simulink model "BatteryTesting100"  (R2022a)
settings: Solver=ode23tb  StartTime=0.0  StopTime=inf  RelTol=1e-3  EnableMultiTasking=on
undefined symbols (not defined in the file or in its folder): Batt, Battery, BatteryCback, BatteryLoadFcn, DC, DOD, gcbh, Q, sps_rtmsupport, spsBatteryLib, Temp
libraries: simulink x7, spsControlledVoltageSourceLib x1, spsCurrentMeasurementLib x1, spsBatteryModel x1, simulink_extras x1, spsSeriesRLCBranchLib x1, spsControlledCurrentSourceLib x1, spspowerguiLib x1
settings Model: Creator=MathWorks  LastModifiedBy=awesomezhao
settings SolverCC: AlgebraicLoopSolver=TrustRegion
settings DataIOCC: LimitDataPoints=on  ReturnWorkspaceOutputs=off
settings OptimizationCC: LifeSpan=inf
settings DebuggingCC: UnconnectedInputMsg=warning  UnconnectedOutputMsg=warning  UnconnectedLineMsg=warning  AllowSymbolicDim=off  SFUnexpectedBacktrackingDiag=warning  SFNoUnconditionalDefaultTransitionDiag=warning  SFExecutionAtInitializationDiag=none  SFMachineParentedDataDiag=warning  ArithmeticOperatorsInVariantConditions=warning
settings HardwareCC: ProdBitPerPointer=32  ProdBitPerSizeT=32  ProdBitPerPtrDiffT=32  ProdLargestAtomicFloat=None  ProdIntDivRoundTo=Undefined  ProdEndianess=Unspecified  ProdWordSize=32  ProdHWDeviceType=32-bit Generic
settings ModelReferenceCC: PropagateSignalLabelsOutOfModel=off
settings SFSimCC: SimUseLocalCustomCode=off  CustomCodeUndefinedFunction=UseInterfaceOnly
settings RTWCC: RTWUseLocalCustomCode=off  DLArmComputeVersion=19.05
settings CodeAppCC: StateflowObjectComments=on
settings GRTTargetCC: TargetLangStandard=C89/C90 (ANSI)
settings ConfigComp: CovMetricSettings=dw  CovSaveCumulativeToWorkspaceVar=on  CovSaveSingleToWorkspaceVar=on  CovExternalEMLEnable=off
settings SimscapeCC: SimscapeNormalizeSystem=off

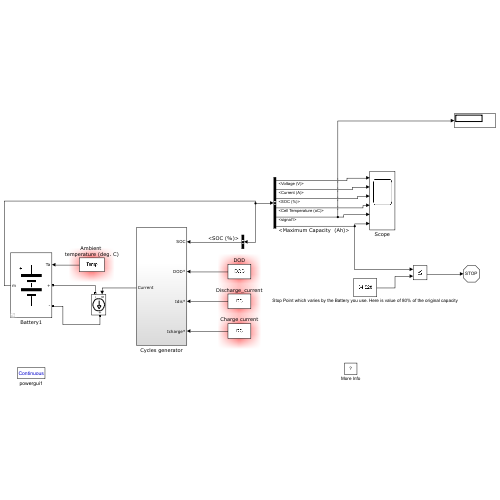
[thumbnail: Simulink's stored preview of the top-level diagram]
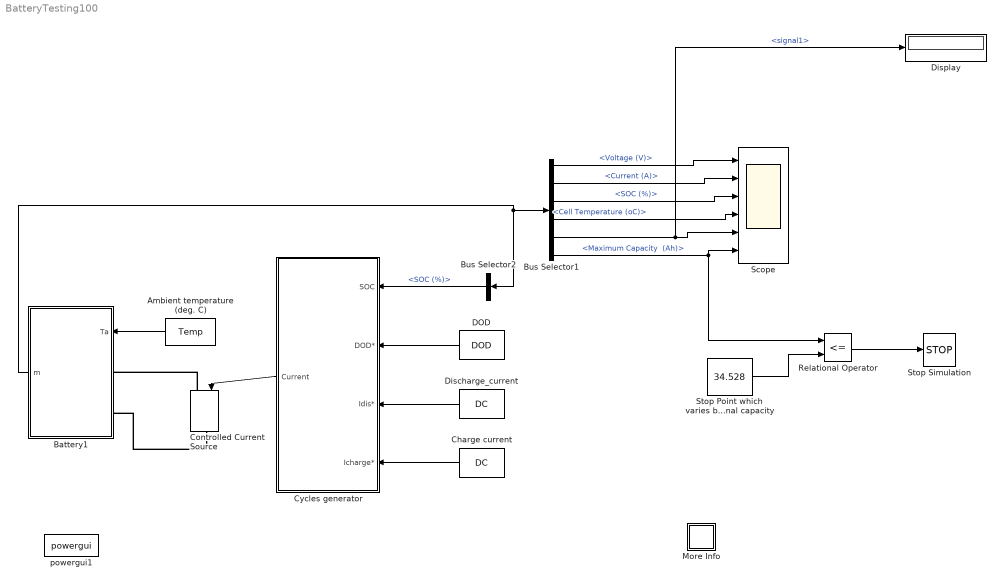
== system BatteryTesting100 ==
  Ambient temperature (deg. C) : Constant  Value=Temp
  Battery1 : Subsystem  AncestorBlock=spsBatteryLib/Battery  DialogController=POWERSYS.PowerSysDialog  LoadFcn=sps_rtmsupport('LoadFcn',gcbh); BatteryLoadFcn(gcb)  InitFcn=BatteryCback(gcb,1)  StartFcn=sps_rtmsupport('StartFcn',gcbh);  StopFcn=sps_rtmsupport('StopFcn',gcbh);  mask(Battery){BatType=Lithium-Ion, ShowTempParam=on, ThermalPreset=12.8V  40Ah  (LiFeMgPO4), ShowAgeParam=on, NomV=12.6, NomQ=40, SOC=100, Batt_Tr=90, PresetModel=off, MaxQ=40, MinV=10.5, FullV=13.8, Dis_rate=20, R=0.015, Normal_OP=30.14, expZone=[13.1          0.5], current=[0.15 1.3 3.25], Units=Ampere-hour, Tci=25, NomT=20, T2=0, MaxQ2=36, FullV2=13, Normal_OP2=11.7, expZone2=[12.67            4], Rca=0.6411, ti=4880, Dp=0, Neq0=0, Tsim=30, Ta1=23, Qeol=40*0.9, Reol=0.0126*1.2, Char_age=[20, 80], Dis_age=[20, 80], N1=1500, N2=10445, N3=1017, N4=1460, Ta2=45, N5=982}
      mask prompts: BatType "Type:"; ShowTempParam "Simulate temperature effects"; ThermalPreset "Use a preset battery:"; ShowAgeParam "Simulate aging effects"; NomV "Nominal voltage (V)"; NomQ "Rated capacity (Ah)"; SOC "Initial state-of-charge (%)"; Batt_Tr "Battery response time (s)"; PresetModel "Determined from the nominal parameters of the battery"; MaxQ "Maximum capacity (Ah)"; MinV "Cut-off Voltage (V)"; FullV "Fully charged voltage (V)"; Dis_rate "Nominal discharge current (A)"; R "Internal resistance (Ohms)"; Normal_OP "Capacity (Ah) at nominal voltage"; expZone "Exponential zone [Voltage (V), Capacity (Ah)]"; current "Discharge current [i1, i2, i3,...] (A)"; Tci "Initial cell temperature (deg. C)"; NomT "Nominal ambient temperature T1 (deg. C)"; T2 "Second ambient temperature T2 (deg. C)"; MaxQ2 "Maximum capacity (Ah)"; FullV2 "Initial discharge voltage (V)"; Normal_OP2 "Voltage at 90% maximum capacity (V)"; expZone2 "Exponential zone [Voltage (V), Capacity (Ah)]"; Rca "Thermal resistance, cell-to-ambient (deg. C/W)"; ti "Thermal time constant, cell-to-ambient (s)"; Dp "Heat loss difference [charge vs. discharge] (W)"; Neq0 "Initial battery age (Equivalent full cycles)"; Tsim "Aging model sampling time (s)"; Ta1 "Ambient temperature Ta1 (deg. C)"; Qeol "Capacity at EOL (End Of Life) (Ah)"; Reol "Internal resistance at EOL (Ohms)"; Char_age "Charge current (nominal, maximum) [Ic (A), Icmax (A)]"; Dis_age "Discharge current (nominal, maximum) [Id (A), Idmax (A)]"; N1 "Cycle life at 100 % DOD, Ic and Id (Cycles)"; N2 "Cycle life at 25 % DOD, Ic and Id (Cycles)"; N3 "Cycle life at 100 % DOD, Ic and Idmax (Cycles)"; N4 "Cycle life at 100 % DOD, Icmax and Id (Cycles)"; Ta2 "Ambient temperature Ta2 (deg. C)"; N5 "Cycle life at 100 % DOD, Ic and Id (Cycles)"
      mask help: Implements a generic battery model for most popular battery types. Temperature and aging (due to cycling) effects can be specified for Lithium-Ion battery type.
      mask init:
      | block = gcb;
      | BatteryCback(block,3)
      | [Batt BT, WantBlockChoice, Ts] = BatteryParam(NomV,NomQ,MaxQ,MinV,FullV,Dis_rate,R,Normal_OP,expZone,block,0);
      | powericon('SetInternalModels','set',block,WantBlockChoice);
      | BatteryCback(block,1);
      settings: CopyFcn=sps_rtmsupport('CopyFcn',gcbh);  DeleteFcn=sps_rtmsupport('DeleteFcn',gcbh);  UndoDeleteFcn=sps_rtmsupport('UndoDeleteFcn',gcbh);  ModelCloseFcn=sps_rtmsupport('ModelCloseFcn',gcbh);  PreSaveFcn=sps_rtmsupport('PreSaveFcn',gcbh);  PostSaveFcn=sps_rtmsupport('PostSaveFcn',gcbh);  NameChangeFcn=sps_rtmsupport('NameChangeFcn',gcbh);  PreCopyFcn=sps_rtmsupport('PreCopyFcn',gcbh);  OpenFcn=sps_rtmsupport('OpenFcn',gcbh, [1,2,3,4,9,18]);  CloseFcn=sps_rtmsupport('CloseFcn',gcbh);  PreDeleteFcn=sps_rtmsupport('PreDeleteFcn',gcbh);
      mask Help: helpview(psbhelp)
      mask TypeOptions BatType: Lead-Acid | Lithium-Ion | Nickel-Cadmium | Nickel-Metal-Hydride
      mask Callback BatType: BatteryCback(gcb,1)
      mask Callback ShowTempParam: BatteryCback(gcb,1)
      mask TypeOptions ThermalPreset: no | 3.3V  2.3Ah  (LiFePO4) | 3.6V  2050mAh   (LiCoO2) | 3.6V  2.0Ah | 3.6V  3.6Ah  (LiNiO2) | 3.6V  4.5Ah | 3.6V  48Ah  (LiNiO2) | 3.7V  4.4Ah | 7.4V  5.4Ah  (LiCoO2) | 11.1V  6600mAh  (LiCoO2) | 12.8V  40Ah  (LiFeMgPO4)
      mask Callback ThermalPreset: BatteryCback(gcb,4)
      mask Callback ShowAgeParam: BatteryCback(gcb,1)
      mask Callback PresetModel: BatteryCback(gcb,1)
      mask TypeOptions Units: Ampere-hour | Time
      mask Callback ti: sps_rtmsupport('parametereditingmodes',gcbh, [1,2,3,4,9,18]);
      mask DialogControl ParameterTabVar0 Prompt: Parameters
      mask DialogControl Tempcontainer Prompt: Temperature
      mask DialogControl Agecontainer Prompt: Aging
      mask DialogControl ParameterTabVar01 Prompt: Discharge
      mask DialogControl Container9 Prompt: Display characteristics
      mask DialogControl PlotButton Prompt: Plot
      mask DialogControl PlotButton Callback: BatteryCback(gcb,0)
      mask DialogControl Temperature Prompt: Temperature
      mask DialogControl Container7 Prompt: Discharge parameters at T2
      mask DialogControl Container8 Prompt: Thermal response and Heat loss
      mask DialogControl Aging Prompt: Aging
      mask DialogControl Container16 Prompt: Aging characteristics at ambient temperature Ta1
      mask DialogControl Container13 Prompt: Aging characteristics at ambient temperature Ta2
  Bus Selector1 : BusSelector  OutputSignals="Voltage (V),Current (A),SOC (%),Cell Temperature (oC),signal1,Maximum Capacity  (Ah)"
  Bus Selector2 : BusSelector  OutputSignals=SOC (%)
  Charge current : Constant  Value=DC
  Controlled Current Source : spsControlledCurrentSourceLib/Controlled Current Source  Initialize=on  Source_Type=AC  Amplitude=0  Phase=0  Frequency=0  Measurements=None
  Cycles generator : Subsystem
  DOD : Constant  Value=DOD
  Discharge_current : Constant  Value=DC
  Display : Display
  More Info : Subsystem
      settings: OpenFcn=showdemo(bdroot(gcb))
      mask Display: disp('?')
  Relational Operator : RelationalOperator  Operator=<=  OutDataTypeStr=boolean  RndMeth=Simplest  InputSameDT=off
  Scope : Scope  NumInputPorts=6
  Stop Point which varies by the Battery you use. Here is value of 80% of the original capacity : Constant  Value=34.528
  Stop Simulation : Stop
  powergui1 : spspowerguiLib/powergui  SimulationMode=Continuous  SampleTime=36  frequency=60  Iterations=50  frequencyindice=0  Pbase=100e6  ErrMax=1e-4  UnitsV=kV  UnitsW=MW  buscounter=0  FunctionMessages=off  echomessages=off  EnableUseOfTLC=off  CurrentSourceSwitches=on  DisableSnubberDevices=off  DisableRonSwitches=off  DisableVfSwitches=off  DisplayEquations=off  AutomaticDiscreteSolvers=off  SolverType=Tustin  Interpol=off  ExternalGateDelay=off  methode=off  Ts=0  x0status=blocks  SPID=off  SwTol=0  HookPort=off  NonlinearTolerance=1e-4  nMaxIteration=100  ContinueOnMaxIteration=off  RestoreLinks=warning  ResistiveCurrentMeasurement=off  Frange=[0:2:500]  Ylog=off  Xlog=on  ShowGrid=off  save=off  variable=ZData  structure=0  ZoomFFT=on  StartTime=0.0  cycles=1  DisplayStyle=1  fundamental=60  FreqAxis=off  MaxFrequency=1000  frequencyindicesteady=1  RmsSteady=1  display=off
  wires:
  Ambient temperature (deg. C)/1 -> Battery1/1(Ta)
  Battery1/1(m) -> Bus Selector2/1, Bus Selector1/1
  Bus Selector1/6 -> Scope/6, Relational Operator/1  "<Maximum Capacity  (Ah)>"
  Cycles generator/1(Current) -> Controlled Current Source/1
  Bus Selector2/1 -> Cycles generator/1(SOC)  "<SOC (%)>"
  Charge current/1 -> Cycles generator/4(Icharge*)
  DOD/1 -> Cycles generator/2(DOD*)
  Discharge_current/1 -> Cycles generator/3(Idis*)
  Stop Point which varies by the Battery you use. Here is value of 80% of the original capacity/1 -> Relational Operator/2
  Relational Operator/1 -> Stop Simulation/1
  Bus Selector1/1 -> Scope/1  "<Voltage (V)>"
  Bus Selector1/2 -> Scope/2  "<Current (A)>"
  Bus Selector1/3 -> Scope/3  "<SOC (%)>"
  Bus Selector1/4 -> Scope/4  "<Cell Temperature (oC)>"
  Bus Selector1/5 -> Display/1, Scope/5  "<signal1>"
  connections:
  Controlled Current Source/LConn1 -- Battery1/LConn1
  Controlled Current Source/RConn1 -- Battery1/LConn2

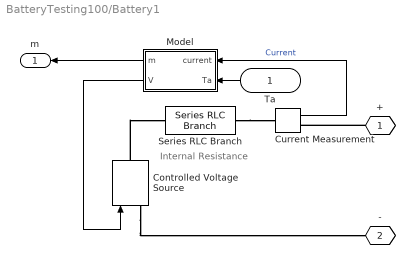
== system BatteryTesting100/Battery1 ==
  note: Internal Resistance
  Ta : Inport
  Controlled Voltage Source : spsControlledVoltageSourceLib/Controlled Voltage Source  Initialize=on  Source_Type=AC  Amplitude=0  Phase=0  Frequency=0  Measurements=None
  Current Measurement : spsCurrentMeasurementLib/Current Measurement  PhasorSimulation=off  OutputType=Complex  PSBequivalent=0
  Model : Subsystem  AncestorBlock=spsBatteryModel/Continuous thermal aging
  Series RLC Branch : spsSeriesRLCBranchLib/Series RLC Branch  LConnTagsString=__new0  RConnTagsString=__new0  BranchType=R  Resistance=Batt.R  Inductance=1e-3  SetiL0=off  InitialCurrent=0  Capacitance=1e-6  Setx0=off  InitialVoltage=0  Measurements=None
  + : PMIOPort  Tag=PMCPort  Side=Left
  - : PMIOPort  Tag=PMCPort  Port=2  Side=Left
  m : Outport  VectorParamsAs1DForOutWhenUnconnected=off
  wires:
  Model/2(V) -> Controlled Voltage Source/1
  Model/1(m) -> m/1
  Current Measurement/1 -> Model/1(current)  "Current"
  Ta/1 -> Model/2(Ta)
  connections:
  +/RConn1 -- Current Measurement/RConn1
  Controlled Voltage Source/LConn1 -- -/RConn1
  Controlled Voltage Source/RConn1 -- Series RLC Branch/LConn1
  Series RLC Branch/RConn1 -- Current Measurement/LConn1

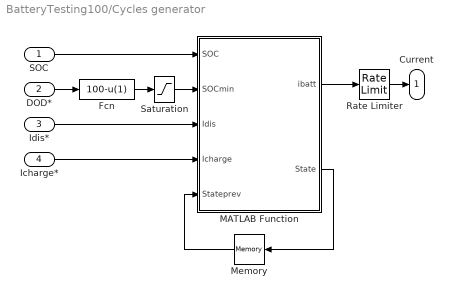
== system BatteryTesting100/Cycles generator ==
  SOC : Inport
  DOD* : Inport  Port=2
  Idis* : Inport  Port=3
  Icharge* : Inport  Port=4
  Fcn : Fcn  Expr=100-u(1)
  MATLAB Function : MATLAB Function  TreatAsAtomicUnit=on
  Memory : Memory  InitialCondition=1
  Rate Limiter : RateLimiter  RisingSlewLimit=1000  FallingSlewLimit=-1000  SampleTimeMode=inherited
  Saturation : Saturate  UpperLimit=98  LowerLimit=1
  Current : Outport  VectorParamsAs1DForOutWhenUnconnected=off
  wires:
  MATLAB Function/1(ibatt) -> Rate Limiter/1
  SOC/1 -> MATLAB Function/1(SOC)
  Memory/1 -> MATLAB Function/5(Stateprev)
  MATLAB Function/2(State) -> Memory/1
  DOD*/1 -> Fcn/1
  Fcn/1 -> Saturation/1
  Saturation/1 -> MATLAB Function/2(SOCmin)
  Idis*/1 -> MATLAB Function/3(Idis)
  Icharge*/1 -> MATLAB Function/4(Icharge)
  Rate Limiter/1 -> Current/1

== system BatteryTesting100/More Info ==

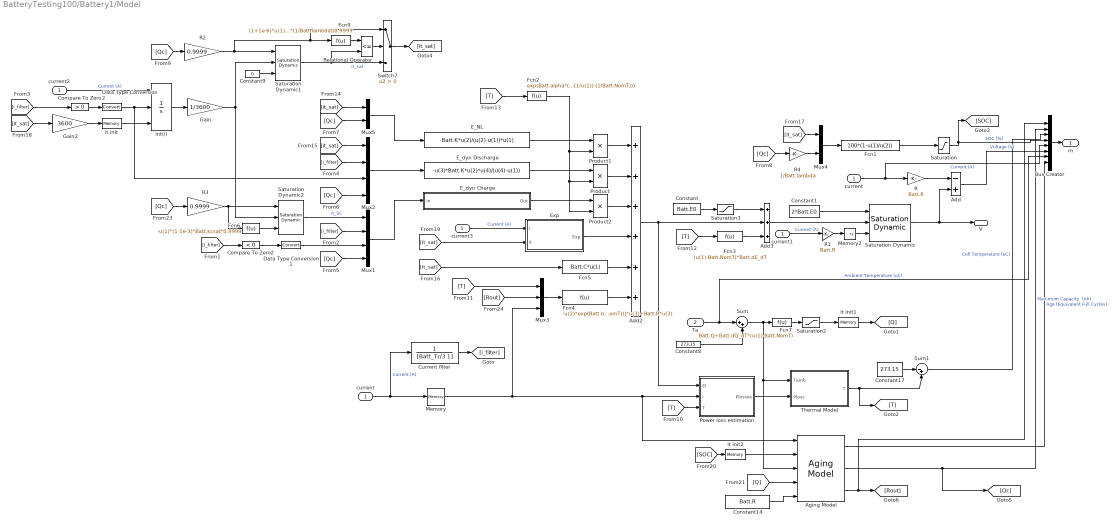
== system BatteryTesting100/Battery1/Model ==
  current : Inport
  Ta : Inport  Port=2
  Add : Sum  Inputs=-+
  Add2 : Sum  Inputs=++++++
  Add3 : Sum  Inputs=+++
  Aging Model : spsBatteryModel/Aging Model  SystemSampleTime=-1  VariantActivationTime=update diagram  Latency=0  AutoFrameSizeCalculation=off
      settings: SourceProductBaseCode=PS
  Bus Creator : BusCreator  Inputs=8
  Compare To Zero : simulink/Logic and Bit Operations/Compare To Zero  relop=>  OutDataTypeStr=uint8
  Compare To Zero2 : simulink/Logic and Bit Operations/Compare To Zero  relop=<  OutDataTypeStr=uint8
  Constant : Constant  Value=Batt.E0
  Constant1 : Constant  Value=2*Batt.E0
  Constant14 : Constant  Value=Batt.R
  Constant17 : Constant  Value=273.15
  Constant8 : Constant  Value=273.15
  Constant9 : Constant  Value=0
  Current filter : TransferFcn  Denominator=[Batt_Tr/3 1]
  Data Type Conversion1 : DataTypeConversion  SaturateOnIntegerOverflow=off  RndMeth=Floor
  Data Type Conversion2 : DataTypeConversion  SaturateOnIntegerOverflow=off  RndMeth=Floor
  E_NL : Fcn  Expr=-Batt.K*u(2)/(u(2)-u(1))*u(1)
  E_dyn Charge : Subsystem
  E_dyn Discharge : Fcn  Expr=-u(3)*Batt.K*u(2)*u(4)/(u(4)-u(1))
  Exp : Subsystem
  Fcn1 : Fcn  Expr=100*(1-u(1)/u(2))
  Fcn2 : Fcn  Expr=exp(Batt.alpha*((1/u(1))-(1/Batt.NomT)))
  Fcn3 : Fcn  Expr=(u(1)-Batt.NomT)*Batt.dE_dT
  Fcn4 : Fcn  Expr=-u(2)*exp(Batt.beta*((1/u(1))-(1/Batt.NomT)))*u(3)+Batt.R*u(3)
  Fcn5 : Fcn  Expr=-Batt.C*u(1)
  Fcn6 : Fcn  Expr=-u(1)*(1-1e-3)*Batt.kcsat*0.9999
  Fcn7 : Fcn  Expr=Batt.Q+Batt.dQ_dT*(u(1)-Batt.NomT)
  Fcn9 : Fcn  Expr=(1+1e-6)*u(1)*(1/Batt.lambda)/0.9999
  Gain : Gain  Gain=1/3600
  Gain2 : Gain  Gain=3600
  Memory : Memory
  Memory2 : Memory  InheritSampleTime=on
  Mux1 : Mux
  Mux2 : Mux
  Mux3 : Mux  Inputs=3
  Mux4 : Mux  Inputs=2
  Mux5 : Mux  Inputs=2
  Power loss estimation : Subsystem
  Product : Product
  Product1 : Product
  Product2 : Product
  R : Gain  Gain=Batt.R
  R1 : Gain  Gain=Batt.R
  R2 : Gain  Gain=0.9999
  R3 : Gain  Gain=0.9999
  R4 : Gain  Gain=1/Batt.lambda
  Relational Operator : RelationalOperator  Operator=<=  RndMeth=Simplest  InputSameDT=off
  Saturation : Saturate  UpperLimit=100  LowerLimit=0
  Saturation Dynamic : simulink/Discontinuities/Saturation Dynamic  OutMin=[]  OutMax=[]  OutDataTypeStr=Inherit: Same as second input  OutDataType=sfix(16)  OutScaling=2^-10  DoSatur=off
  Saturation Dynamic1 : simulink/Discontinuities/Saturation Dynamic  OutMin=[]  OutMax=[]  OutDataTypeStr=Inherit: Same as second input  OutDataType=sfix(16)  OutScaling=2^-10  DoSatur=off
  Saturation Dynamic2 : simulink/Discontinuities/Saturation Dynamic  OutMin=[]  OutMax=[]  OutDataTypeStr=Inherit: Same as second input  OutDataType=sfix(16)  OutScaling=2^-10  DoSatur=off
  Saturation2 : Saturate  UpperLimit=max(NomQ,Batt.Q)  LowerLimit=0
  Saturation3 : Saturate  UpperLimit=Batt.Va-Batt.dE_dT*(Batt.Tci-Batt.NomT)-Batt.A  LowerLimit=-inf
  Sum : Sum  Inputs=|++
  Sum1 : Sum  Inputs=|-+
  Switch7 : Switch  Criteria=u2 > Threshold  SaturateOnIntegerOverflow=off  InputSameDT=off
  Thermal Model : Subsystem  VariantControl=Continuous
  "current " : InportShadow
  current1 : InportShadow
  current2 : InportShadow
  current3 : InportShadow
  int(i) : Integrator  ExternalReset=rising  InitialConditionSource=external  InitialCondition=(1-SOC/100)*Q*3600  LimitOutput=on  UpperSaturationLimit=Batt.Qmax*3600
  it init : Memory  InitialCondition=(1-SOC/100)*Batt.Q*(1/Batt.lambda)*3600
  it init1 : Memory  InitialCondition=Batt.Q
  it init2 : Memory  InitialCondition=SOC
  m : Outport  VectorParamsAs1DForOutWhenUnconnected=off
  V : Outport  Port=2  VectorParamsAs1DForOutWhenUnconnected=off
  wires:
  Sum1/1 -> Bus Creator/3  "Cell Temperature (oC)"
  Thermal Model/1(T) -> [T], Sum1/2
  Constant17/1 -> Sum1/1
  Relational Operator/1 -> Switch7/2
  Fcn9/1 -> Relational Operator/1
  Switch7/1 -> [it_sat]
  R2/1 -> Saturation Dynamic1/1, Fcn9/1, Switch7/1
  Saturation Dynamic1/1 -> Switch7/3, Relational Operator/2  "it_sat"
  R1/1 -> Memory2/1
  Memory2/1 -> Saturation Dynamic/3
  current1/1 -> R1/1  "Current (A)"
  Constant9/1 -> Saturation Dynamic1/3
  Gain/1 -> Saturation Dynamic2/2, Saturation Dynamic1/2
  it init2/1 -> Aging Model/2
  [Rout] -> Mux3/2
  Aging Model/3 -> Bus Creator/1, [Rout]
  Constant14/1 -> Aging Model/5
  Aging Model/2 -> [Qc], Bus Creator/2  "Maximum Capacity  (Ah)"
  [Q] -> Aging Model/4
  [SOC] -> it init2/1
  [Qc] -> Mux5/2
  Saturation Dynamic/1 -> Add/2, V/1
  Saturation/1 -> [SOC], Bus Creator/4  "SOC (%)"
  R4/1 -> Mux4/2
  [T] -> Power loss estimation/3(T)
  Add2/1 -> Add3/2, Power loss estimation/1(El)
  R3/1 -> Saturation Dynamic2/1, Fcn6/1
  [Qc] -> R3/1
  [it_sat] -> Exp/2(it)
  [it_sat] -> Gain2/1
  [it_sat] -> Mux4/1
  [it_sat] -> Fcn5/1
  [it_sat] -> Mux2/1
  [it_sat] -> Mux5/1
  [T] -> Fcn2/1
  [T] -> Fcn3/1
  [T] -> Mux3/1
  [Qc] -> R2/1
  [Qc] -> R4/1
  [Qc] -> Mux2/4
  [Qc] -> Mux1/4
  it init1/1 -> [Q]
  [i_filter] -> Mux2/2
  [i_filter] -> Compare To Zero/1
  [i_filter] -> Mux1/2
  [i_filter] -> Compare To Zero2/1
  Current filter/1 -> [i_filter]
  "current "/1 -> Current filter/1, Memory/1  "Current (A)"
  current3/1 -> Exp/1(i)  "Current (A)"
  current2/1 -> int(i)/1  "Current (A)"
  Saturation2/1 -> it init1/1
  Saturation3/1 -> Add3/1
  Fcn7/1 -> Saturation2/1
  Sum/1 -> Fcn7/1, Thermal Model/1(Tamb), Aging Model/3
  Fcn6/1 -> Saturation Dynamic2/3
  Fcn3/1 -> Add3/3
  Mux5/1 -> E_NL/1
  Mux4/1 -> Fcn1/1
  Constant8/1 -> Sum/2
  Ta/1 -> Bus Creator/7, Sum/1  "Ambient Temperature (oC)"
  Fcn5/1 -> Add2/5
  Product2/1 -> Add2/3
  E_dyn Charge/1(Out) -> Product2/1
  Mux3/1 -> Fcn4/1
  Fcn4/1 -> Add2/6
  Fcn2/1 -> Product1/2, Product/2, Product2/2
  Power loss estimation/1(Plosses) -> Thermal Model/2(Ploss)
  Memory/1 -> Power loss estimation/2(i), Aging Model/1, Mux3/3
  Product1/1 -> Add2/1
  E_NL/1 -> Product1/1
  Product/1 -> Add2/2
  E_dyn Discharge/1 -> Product/1
  Add3/1 -> Saturation Dynamic/2
  Constant1/1 -> Saturation Dynamic/1
  Saturation Dynamic2/1 -> Mux1/1  "it_SC"
  Data Type Conversion1/1 -> Mux1/3
  Exp/1(Exp) -> Add2/4
  Gain2/1 -> it init/1
  Data Type Conversion2/1 -> int(i)/2, Mux2/3
  Compare To Zero2/1 -> Data Type Conversion1/1
  Compare To Zero/1 -> Data Type Conversion2/1
  it init/1 -> int(i)/3
  Mux1/1 -> E_dyn Charge/1(In)
  Constant/1 -> Saturation3/1
  Mux2/1 -> E_dyn Discharge/1
  Bus Creator/1 -> m/1
  R/1 -> Add/1
  Add/1 -> Bus Creator/6  "Voltage (V)"
  Fcn1/1 -> Saturation/1
  int(i)/1 -> Gain/1
  current/1 -> R/1, Bus Creator/5  "Current (A)"
  Aging Model/1 -> Bus Creator/8  "Age (Equivalent Full Cycles)"

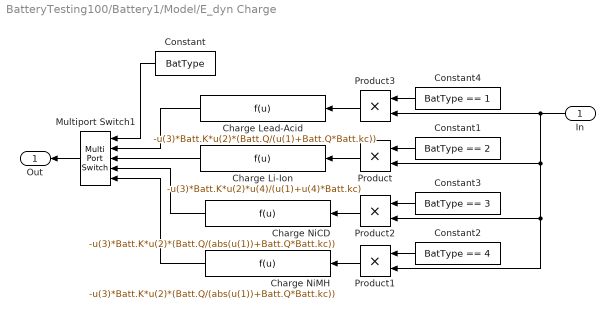
== system BatteryTesting100/Battery1/Model/E_dyn Charge ==
  In : Inport
  Charge Lead-Acid : Fcn  Expr=-u(3)*Batt.K*u(2)*(Batt.Q/(u(1)+Batt.Q*Batt.kc))
  Charge Li-Ion : Fcn  Expr=-u(3)*Batt.K*u(2)*u(4)/(u(1)+u(4)*Batt.kc)
  Charge NiCD : Fcn  Expr=-u(3)*Batt.K*u(2)*(Batt.Q/(abs(u(1))+Batt.Q*Batt.kc))
  Charge NiMH : Fcn  Expr=-u(3)*Batt.K*u(2)*(Batt.Q/(abs(u(1))+Batt.Q*Batt.kc))
  Constant : Constant  Value=BatType
  Constant1 : Constant  Value=BatType == 2  OutDataTypeStr=double
  Constant2 : Constant  Value=BatType == 4  OutDataTypeStr=double
  Constant3 : Constant  Value=BatType == 3  OutDataTypeStr=double
  Constant4 : Constant  Value=BatType == 1  OutDataTypeStr=double
  Multiport Switch1 : MultiPortSwitch  Inputs=4  SaturateOnIntegerOverflow=off  InputSameDT=off
  Product{,1..3} (4 alike) : Product  RndMeth=Zero
  Out : Outport  VectorParamsAs1DForOutWhenUnconnected=off
  wires:
  Constant4/1 -> Product3/1
  Product3/1 -> Charge Lead-Acid/1
  Constant3/1 -> Product2/1
  Product2/1 -> Charge NiCD/1
  Constant2/1 -> Product1/1
  Product1/1 -> Charge NiMH/1
  Constant1/1 -> Product/1
  Product/1 -> Charge Li-Ion/1
  In/1 -> Product2/2, Product1/2, Product/2, Product3/2
  Constant/1 -> Multiport Switch1/1
  Charge Lead-Acid/1 -> Multiport Switch1/2
  Charge NiCD/1 -> Multiport Switch1/4
  Charge NiMH/1 -> Multiport Switch1/5
  Charge Li-Ion/1 -> Multiport Switch1/3
  Multiport Switch1/1 -> Out/1

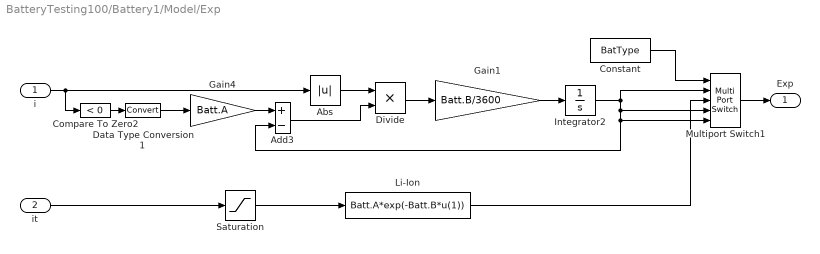
== system BatteryTesting100/Battery1/Model/Exp ==
  i : Inport
  it : Inport  Port=2
  Abs : Abs  SaturateOnIntegerOverflow=off
  Add3 : Sum  Inputs=+-
  Compare To Zero2 : simulink/Logic and Bit Operations/Compare To Zero  relop=<  OutDataTypeStr=uint8
  Constant : Constant  Value=BatType
  Data Type Conversion1 : DataTypeConversion  SaturateOnIntegerOverflow=off  RndMeth=Floor
  Divide : Product  Inputs=**
  Gain1 : Gain  Gain=Batt.B/3600
  Gain4 : Gain  Gain=Batt.A
  Integrator2 : Integrator  InitialCondition=Batt.A*exp(-Batt.B*(1-SOC/100)*Batt.Q)
  Li-Ion : Fcn  Expr=Batt.A*exp(-Batt.B*u(1))
  Multiport Switch1 : MultiPortSwitch  Inputs=4  SaturateOnIntegerOverflow=off  InputSameDT=off
  Saturation : Saturate  UpperLimit=Batt.Qmax*(1/Batt.lambda)  LowerLimit=-inf
  Exp : Outport  VectorParamsAs1DForOutWhenUnconnected=off
  wires:
  Saturation/1 -> Li-Ion/1
  Data Type Conversion1/1 -> Gain4/1
  Compare To Zero2/1 -> Data Type Conversion1/1
  Multiport Switch1/1 -> Exp/1
  Li-Ion/1 -> Multiport Switch1/3
  it/1 -> Saturation/1
  Constant/1 -> Multiport Switch1/1
  i/1 -> Compare To Zero2/1, Abs/1
  Gain1/1 -> Integrator2/1
  Add3/1 -> Divide/2
  Abs/1 -> Divide/1
  Divide/1 -> Gain1/1
  Gain4/1 -> Add3/1
  Integrator2/1 -> Multiport Switch1/5, Add3/2, Multiport Switch1/4, Multiport Switch1/2

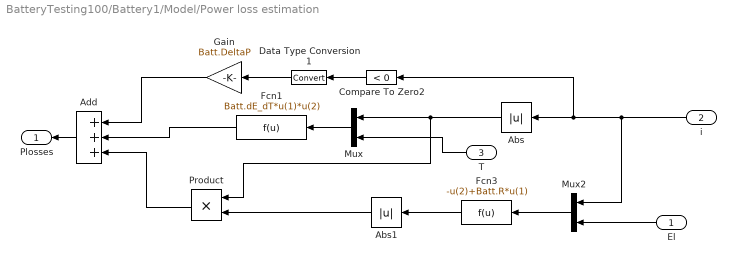
== system BatteryTesting100/Battery1/Model/Power loss estimation ==
  El : Inport
  i : Inport  Port=2
  T : Inport  Port=3
  Abs : Abs  SaturateOnIntegerOverflow=off
  Abs1 : Abs  SaturateOnIntegerOverflow=off
  Add : Sum  Inputs=+++
  Compare To Zero2 : simulink/Logic and Bit Operations/Compare To Zero  relop=<  OutDataTypeStr=uint8
  Data Type Conversion1 : DataTypeConversion  SaturateOnIntegerOverflow=off  RndMeth=Floor
  Fcn1 : Fcn  Expr=Batt.dE_dT*u(1)*u(2)
  Fcn3 : Fcn  Expr=-u(2)+Batt.R*u(1)
  Gain : Gain  Gain=Batt.DeltaP
  Mux : Mux  Inputs=2
  Mux2 : Mux  Inputs=2
  Product : Product
  Plosses : Outport  VectorParamsAs1DForOutWhenUnconnected=off
  wires:
  Gain/1 -> Add/1
  Data Type Conversion1/1 -> Gain/1
  Compare To Zero2/1 -> Data Type Conversion1/1
  Fcn1/1 -> Add/2
  Product/1 -> Add/3
  Mux2/1 -> Fcn3/1
  Fcn3/1 -> Abs1/1
  El/1 -> Mux2/2
  Abs1/1 -> Product/2
  Abs/1 -> Product/1, Mux/1
  Mux/1 -> Fcn1/1
  Add/1 -> Plosses/1
  T/1 -> Mux/2
  i/1 -> Mux2/1, Abs/1, Compare To Zero2/1

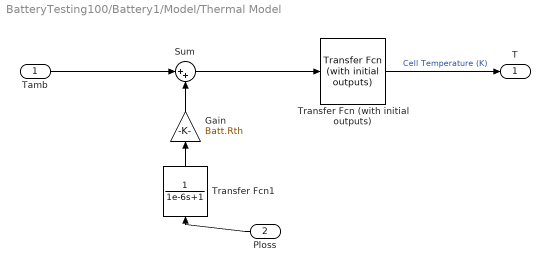
== system BatteryTesting100/Battery1/Model/Thermal Model ==
  Tamb : Inport
  Ploss : Inport  Port=2
  Gain : Gain  Gain=Batt.Rth
  Sum : Sum  Inputs=|++
  Transfer Fcn (with initial outputs) : simulink_extras/Additional Linear/Transfer Fcn (with initial outputs)  N=[1]  D="[Batt.tc  1]"  Y0=Batt.Tci  U0=0
  Transfer Fcn1 : TransferFcn  Denominator=[1e-6 1]
  T : Outport  VectorParamsAs1DForOutWhenUnconnected=off
  wires:
  Sum/1 -> Transfer Fcn (with initial outputs)/1
  Gain/1 -> Sum/2
  Ploss/1 -> Transfer Fcn1/1
  Transfer Fcn (with initial outputs)/1 -> T/1  "Cell Temperature (K)"
  Transfer Fcn1/1 -> Gain/1
  Tamb/1 -> Sum/1

== matlab function BatteryTesting100/Cycles generator/MATLAB Function ==
  data: SOC input; SOCmin input; Idis input; Icharge input; ibatt output; Stateprev input; State output
function [ibatt,State] = fcn(SOC,SOCmin,Idis,Icharge,Stateprev)
%#codegen
State=Stateprev;
if(Stateprev==1 && SOC<=SOCmin)
    State=0;
end
if(Stateprev==0 && SOC>=99)
    State=1;
end
if (Stateprev==1)
    ibatt=Idis;
else
    ibatt=-Icharge;
end
